simulink model "miss_simulink02_basic"  (R2024b)
settings: Solver=VariableStepAuto  StartTime=0.0  StopTime=10.0  RelTol=1e-3
settings Model: Creator=user  LastModifiedBy=user

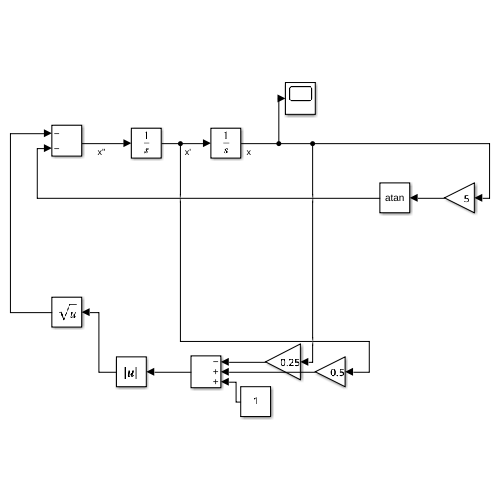
[thumbnail: Simulink's stored preview of the top-level diagram]
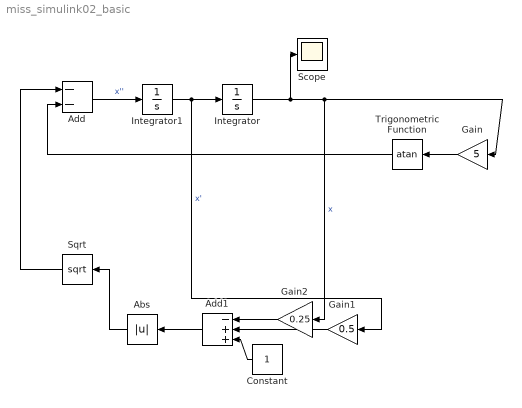
== system miss_simulink02_basic ==
  Abs : Abs  SaturateOnIntegerOverflow=off
  Add : Sum  Inputs=--
  Add1 : Sum  Inputs=-++
  Constant : Constant
  Gain : Gain  Gain=5
  Gain1 : Gain  Gain=0.5
  Gain2 : Gain  Gain=0.25
  Integrator : Integrator
  Integrator1 : Integrator
  Scope : Scope
  Sqrt : Sqrt
  Trigonometric Function : Trigonometry  Operator=atan
  wires:
  Integrator1/1 -> Gain1/1, Integrator/1  "x'"
  Add/1 -> Integrator1/1  "x''"
  Integrator/1 -> Scope/1, Gain2/1, Gain/1  "x"
  Gain/1 -> Trigonometric Function/1
  Trigonometric Function/1 -> Add/2
  Gain1/1 -> Add1/2
  Gain2/1 -> Add1/1
  Constant/1 -> Add1/3
  Add1/1 -> Abs/1
  Abs/1 -> Sqrt/1
  Sqrt/1 -> Add/1
